simulink model "q_1"  (R2020a)
settings: Solver=VariableStepAuto  StartTime=0.0  StopTime=10.0  RelTol=1e-3
values from neighbouring files (symbols this model uses):
  b = 50    [mech.mat]
  F = [-1.08804222178 1.82589050146 -1.97606324819 1.49022632096 -0.524749707408 -0.609621242204 1.54778136312 -1.98777730785 1.7879933272 -1.01273128222 -0.0884853561701 1.16122236842 ... (100 elements, 1x100)]    [mech.mat]
  k1 = 50    [mech.mat]
  k12 = 1000    [mech.mat]
  m1 = 100    [mech.mat]
  m2 = 0.25    [mech.mat]
settings Model: Creator=Admin  LastModifiedBy=Admin

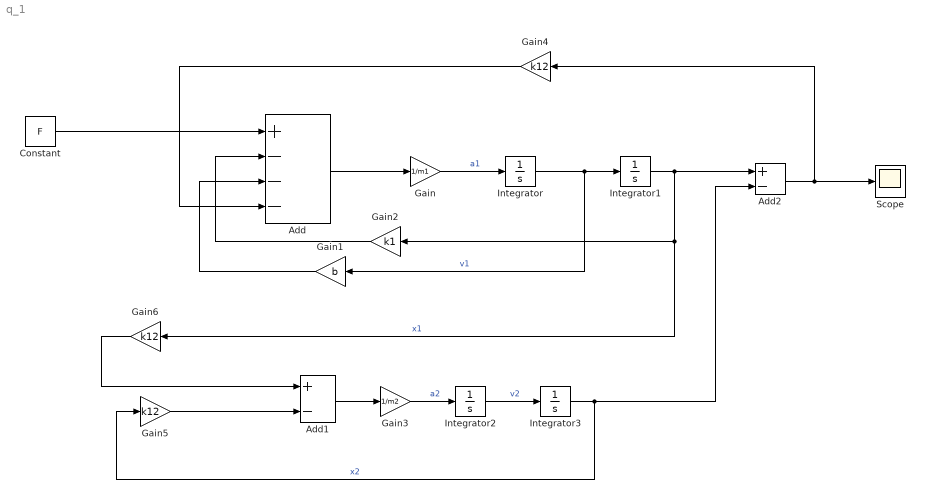
== system q_1 ==
  Add : Sum  Inputs=+---
  Add1 : Sum  Inputs=+-
  Add2 : Sum  Inputs=+-
  Constant : Constant  Value=F
  Gain : Gain  Gain=1/m1
  Gain1 : Gain  Gain=b
  Gain2 : Gain  Gain=k1
  Gain3 : Gain  Gain=1/m2
  Gain4 : Gain  Gain=k12
  Gain5 : Gain  Gain=k12
  Gain6 : Gain  Gain=k12
  Integrator{,1..3} (4 alike) : Integrator
  Scope : Scope
  wires:
  Gain/1 -> Integrator/1  "a1"
  Integrator/1 -> Gain1/1, Integrator1/1  "v1"
  Add/1 -> Gain/1
  Integrator1/1 -> Gain6/1, Gain2/1, Add2/1  "x1"
  Constant/1 -> Add/1
  Gain1/1 -> Add/3
  Gain2/1 -> Add/2
  Add1/1 -> Gain3/1
  Gain3/1 -> Integrator2/1  "a2"
  Integrator2/1 -> Integrator3/1  "v2"
  Gain4/1 -> Add/4
  Gain5/1 -> Add1/2
  Integrator3/1 -> Add2/2, Gain5/1  "x2"
  Add2/1 -> Gain4/1, Scope/1
  Gain6/1 -> Add1/1
